simulink subsystem "Motor"  (R2024a)
settings: Solver=VariableStepAuto  StartTime=0.0  StopTime=10.0  RelTol=1e-3
undefined symbols (not defined in the file or in its folder): useGenerator
settings Model: Creator=20192648  LastModifiedBy=20192648

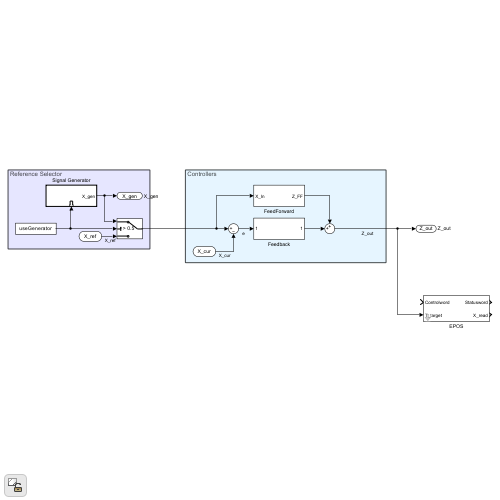
[thumbnail: Simulink's stored preview of the top-level diagram]
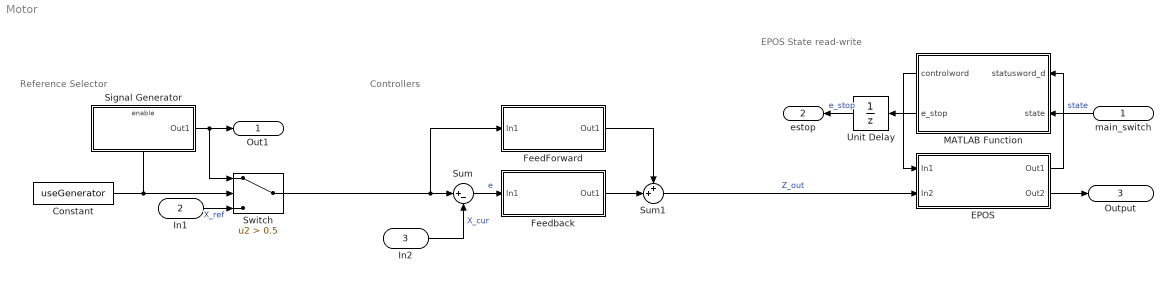
== system Motor ==
  note: EPOS State read-write
  note: Controllers
  note: Reference Selector
  main_switch : Inport
  In1 : Inport  Port=2
  In2 : Inport  Port=3
  Constant : Constant  Value=useGenerator
  EPOS : Subsystem  mask{link_id=1, operating_mode=CyclicSynchronousTorque}
      mask prompts: link_id "link id > 0"; operating_mode "Operating mode of the drive"
      mask TypeOptions operating_mode: CyclicSynchronousPosition | CyclicSynchronousVelocity | CyclicSynchronousTorque
  FeedForward : Subsystem
  Feedback : Subsystem
  MATLAB Function : MATLAB Function  TreatAsAtomicUnit=on
  Signal Generator : Subsystem  TreatAsAtomicUnit=on
  Sum : Sum  Inputs=|+-
  Sum1 : Sum  Inputs=++|
  Switch : Switch  Criteria=u2 > Threshold  Threshold=0.5  SaturateOnIntegerOverflow=off  InputSameDT=off
  Unit Delay : UnitDelay  SampleTime=-1  HasFrameUpgradeWarning=on
  Out1 : Outport  SignalName=X_gen
  estop : Outport  Port=2  SignalName=Z_out
  Output : Outport  Port=3
  wires:
  In2/1 -> Sum/2  "X_cur"
  Signal Generator/1(Out1) -> Out1/1, Switch/1
  Feedback/1(Out1) -> Sum1/2
  Sum/1 -> Feedback/1(In1)  "e"
  FeedForward/1(Out1) -> Sum1/1
  Sum1/1 -> EPOS/2(In2)  "Z_out"
  Constant/1 -> Switch/2, Signal Generator/Enable
  In1/1 -> Switch/3  "X_ref"
  Switch/1 -> Sum/1, FeedForward/1(In1)
  EPOS/1(Out1) -> MATLAB Function/1(statusword_d)
  MATLAB Function/1(controlword) -> EPOS/1(In1)
  MATLAB Function/2(e_stop) -> Unit Delay/1
  EPOS/2(Out2) -> Output/1
  main_switch/1 -> MATLAB Function/2(state)  "state"
  Unit Delay/1 -> estop/1  "e_stop"

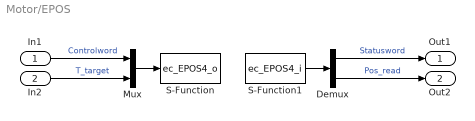
== system Motor/EPOS ==
  In1 : Inport
  In2 : Inport  Port=2
  Demux : Demux  Outputs=2
  Mux : Mux  Inputs=2
  S-Function : S-Function  FunctionName=ec_EPOS4_o  Parameters=link_id  SFunctionDeploymentMode=off  EnableBusSupport=off
  S-Function1 : S-Function  FunctionName=ec_EPOS4_i  Parameters=link_id operating_mode  SFunctionDeploymentMode=off  EnableBusSupport=off
  Out1 : Outport
  Out2 : Outport  Port=2
  wires:
  Demux/2 -> Out2/1  "Pos_read"
  Demux/1 -> Out1/1  "Statusword"
  S-Function1/1 -> Demux/1
  Mux/1 -> S-Function/1
  In2/1 -> Mux/2  "T_target"
  In1/1 -> Mux/1  "Controlword"

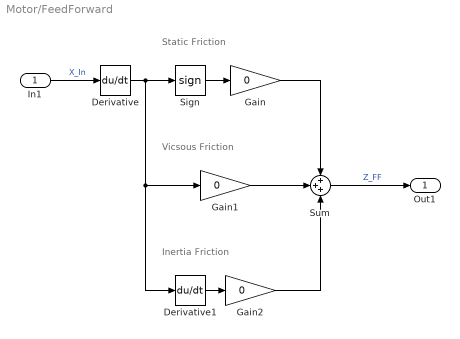
== system Motor/FeedForward ==
  note: Static Friction
  note: Vicsous Friction
  note: Inertia Friction
  In1 : Inport
  Derivative : Derivative
  Derivative1 : Derivative
  Gain : Gain  Gain=0
  Gain1 : Gain  Gain=0
  Gain2 : Gain  Gain=0
  Sign : Signum
  Sum : Sum  Inputs=+++
  Out1 : Outport
  wires:
  Sum/1 -> Out1/1  "Z_FF"
  Gain2/1 -> Sum/3
  Gain1/1 -> Sum/2
  Gain/1 -> Sum/1
  Derivative1/1 -> Gain2/1
  Derivative/1 -> Sign/1, Derivative1/1, Gain1/1
  Sign/1 -> Gain/1
  In1/1 -> Derivative/1  "X_In"

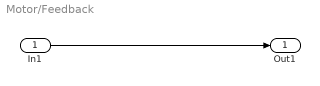
== system Motor/Feedback ==
  In1 : Inport
  Out1 : Outport
  wires:
  In1/1 -> Out1/1

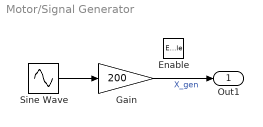
== system Motor/Signal Generator ==
  Enable : EnablePort
  Gain : Gain  Gain=200
  Sine Wave : Sin  SampleTime=0
  Out1 : Outport
  wires:
  Gain/1 -> Out1/1  "X_gen"
  Sine Wave/1 -> Gain/1

== matlab function Motor/MATLAB Function ==
  data: statusword_d input; controlword output; state input; e_stop output
function [controlword, e_stop] = fcn(statusword_d, state)

%% === Statusword bits ===
BIT_READY_TO_SWITCH_ON    = uint16(1);
BIT_SWITCHED_ON           = uint16(2);
BIT_OPERATION_ENABLED     = uint16(4);
BIT_FAULT                 = uint16(8);
BIT_QUICK_STOP            = uint16(32);
BIT_SWITCH_ON_DISABLED    = uint16(64);

%% === Controlwords ===
CTRL_SHUTDOWN     = uint16(6);
CTRL_SWITCH_ON    = uint16(7);
CTRL_ENABLE_OP    = uint16(15);
CTRL_QUICK_STOP   = uint16(2);
CTRL_FAULT_RESET  = uint16(128);

%% Convert raw statusword
statusword = uint16(statusword_d);

%% === Correct hardware E-STOP detection ===
qs_active = bitand(statusword, BIT_QUICK_STOP) ~= 0;

% Hardware estop only if QS active and YOU did NOT command Quick_Stop
e_stop = qs_active && state ~= State_Transition_TableModeType.Quick_Stopping;

%% === Priority 1: Hardware ESTOP ===
if e_stop
    controlword = double(CTRL_SHUTDOWN);
    return;
end

%% === Priority 2: Logical STOP from supervisor ===
if state == State_Transition_TableModeType.Stopped
    controlword = double(CTRL_SHUTDOWN);
    return;
end

%% === Priority 3: Idle → shutdown ===
if state == State_Transition_TableModeType.Idle
    controlword = double(CTRL_SHUTDOWN);
    return;
end

%% === Priority 4: Quick stop request ===
if state == State_Transition_TableModeType.Quick_Stopping
    controlword = double(CTRL_QUICK_STOP);
    return;
end

%% === Priority 5: Running → follow CiA-402 state machine ===
if state == State_Transition_TableModeType.Running

    if bitand(statusword, BIT_FAULT) ~= 0
        controlword = double(CTRL_FAULT_RESET);

    elseif bitand(statusword, BIT_READY_TO_SWITCH_ON) ~= 0 && ...
           bitand(statusword, BIT_SWITCHED_ON) == 0
        controlword = double(CTRL_SWITCH_ON);

    elseif bitand(statusword, BIT_SWITCHED_ON) ~= 0 && ...
           bitand(statusword, BIT_OPERATION_ENABLED) == 0
        controlword = double(CTRL_ENABLE_OP);

    elseif bitand(statusword, BIT_OPERATION_ENABLED) ~= 0
        controlword = double(CTRL_ENABLE_OP);

    else
        controlword = double(CTRL_SHUTDOWN);
    end

    return;
end

%% === Fallback ===
controlword = double(CTRL_SHUTDOWN);
end
